simulink model "chart"  (R2020a)
settings: Solver=VariableStepAuto  StartTime=0.0  StopTime=2  RelTol=1e-3
model workspace: external: MATLAB File C:\Users\Dat Nguyen\Documents\GitHub\MAE-162E\Simple_Robot\simple_robot_DataFile.m (data not in the file)
settings Model: Creator=sgess  LastModifiedBy=David

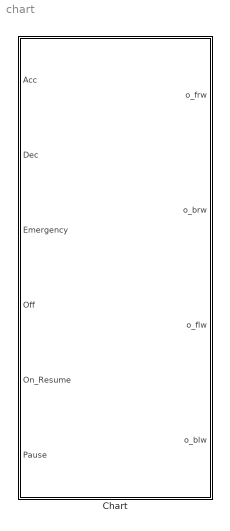
== system chart ==
  Chart : Stateflow chart  TreatAsAtomicUnit=on

== stateflow chart chart/Chart ==
  state On
    state Running
      entry:
      o_flw=-state_speed;
      o_frw=state_speed;
      o_blw=-state_speed;
      o_brw=state_speed;
    state Pause
      entry:
      o_flw=0;
      o_frw=0;
      o_blw=0;
      o_brw=0;
    state Acc
      entry:
      state_speed=state_speed+5;
    state Dec
      entry:
      state_speed=state_speed-5;
    (default) -> Running
    Pause -> Running : [Pause == 0 && On_Resume ==1]
    Running -> Pause [order 1] : [Pause == 1]
    Running -> Acc [order 2] : [Acc==1 && Dec == 0]
    Running -> Acc [order 3] : [Acc == 0]
    Running -> Dec [order 4] : [Dec==1 && Acc==0]
    Running -> Dec [order 5] : [Dec==0]
  state Off
    entry:
    state_speed=0;
    o_flw=0;
    o_frw=0;
    o_blw=0;
    o_brw=0;
  (default) -> Off
  Off -> On : [On_Resume == 1]
  On -> Off : [Emergency || Off == 1]
  data: o_frw output; o_brw output; o_flw output; o_blw output; Acc input; Dec input; Emergency input; Off input; On_Resume input; Pause input; state_speed local
